simulink model "setup_model"  (R2024b)
settings: Solver=FixedStepAuto  StartTime=0.0  StopTime=t_end_s  FixedStep=t_sim_s  RelTol=1e-3
undefined symbols (not defined in the file or in its folder): duty_amp, omega_e_radps
settings Model: Creator=sung0058  LastModifiedBy=mokht029
settings OptimizationCC: DefaultParameterBehavior=Inlined  EnhancedBackFolding=on  PassReuseOutputArgsAs=Individual arguments  ZeroExternalMemoryAtStartup=off  ZeroInternalMemoryAtStartup=off  OptimizeBlockOrder=speed  DifferentSizesBufferReuse=on  OptimizationCustomize=off  EfficientTunableParamExpr=on
settings DebuggingCC: ParameterTunabilityLossMsg=error
settings SFSimCC: MATLABDynamicMemAlloc=off
settings RTWCC: Description=Embedded Coder  SystemTargetFile=ert.tlc  GenCodeOnly=on  TemplateMakefile=ert_default_tmf
settings CodeAppCC: ForceParamTrailComments=on  IgnoreCustomStorageClasses=off  OperatorAnnotations=on  SimulinkDataObjDesc=on  SFDataObjDesc=on  InsertBlockDesc=on
settings ERTTargetCC: TargetLangStandard=C99 (ISO)  ERTCustomFileTemplate=example_file_process.tlc

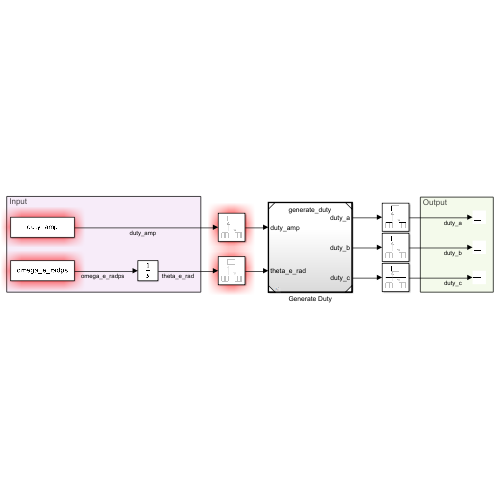
[thumbnail: Simulink's stored preview of the top-level diagram]
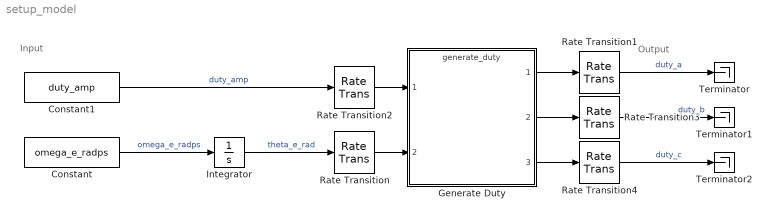
== system setup_model ==
  note: Output
  note: Input
  Constant : Constant  Value=omega_e_radps
  Constant1 : Constant  Value=duty_amp
  Generate Duty : ModelReference  ModelNameDialog=generate_duty.slx  SimulationMode=Normal  ModelReferenceVersion=1.3
  Integrator : Integrator
  Rate Transition : RateTransition  OutPortSampleTime=t_s_s
  Rate Transition1 : RateTransition
  Rate Transition2 : RateTransition  OutPortSampleTime=t_s_s
  Rate Transition3 : RateTransition
  Rate Transition4 : RateTransition
  Terminator : Terminator
  Terminator1 : Terminator
  Terminator2 : Terminator
  wires:
  Constant/1 -> Integrator/1  "omega_e_radps"
  Integrator/1 -> Rate Transition/1  "theta_e_rad"
  Constant1/1 -> Rate Transition2/1  "duty_amp"
  Rate Transition1/1 -> Terminator/1  "duty_a"
  Rate Transition3/1 -> Terminator1/1  "duty_b"
  Rate Transition4/1 -> Terminator2/1  "duty_c"
  Rate Transition2/1 -> Generate Duty/1
  Rate Transition/1 -> Generate Duty/2
  Generate Duty/1 -> Rate Transition1/1
  Generate Duty/2 -> Rate Transition3/1
  Generate Duty/3 -> Rate Transition4/1
